simulink model "engine_test_bed"  (R2022b)
settings: Solver=FixedStepAuto  StartTime=0.0  StopTime=250  FixedStep=1e-3  RelTol=1e-3
InitFcn:
  | lqr_cont;
  | ref_calc;
values from neighbouring files (symbols this model uses):
  rpm = ones(1,3)    [ref_calc.m]
  torque = ones(1,3)    [ref_calc.m]
undefined symbols (not defined in the file or in its folder): K
settings Model: Creator=Cemil  LastModifiedBy=Cemil
settings SolverCC: AlgebraicLoopSolver=TrustRegion
settings DebuggingCC: UnconnectedInputMsg=warning  UnconnectedOutputMsg=warning  UnconnectedLineMsg=warning  SFMachineParentedDataDiag=warning
settings HardwareCC: ProdHWDeviceType=AMD->x86-64 (Windows64)
settings ModelReferenceCC: EnableRefExpFcnMdlSchedulingChecks=on
settings RTWCC: DLArmComputeVersion=19.05

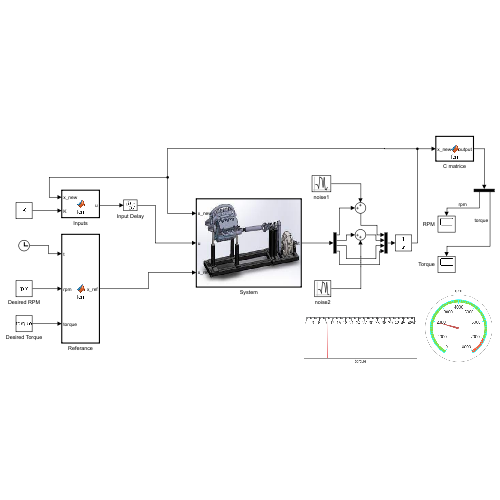
[thumbnail: Simulink's stored preview of the top-level diagram]
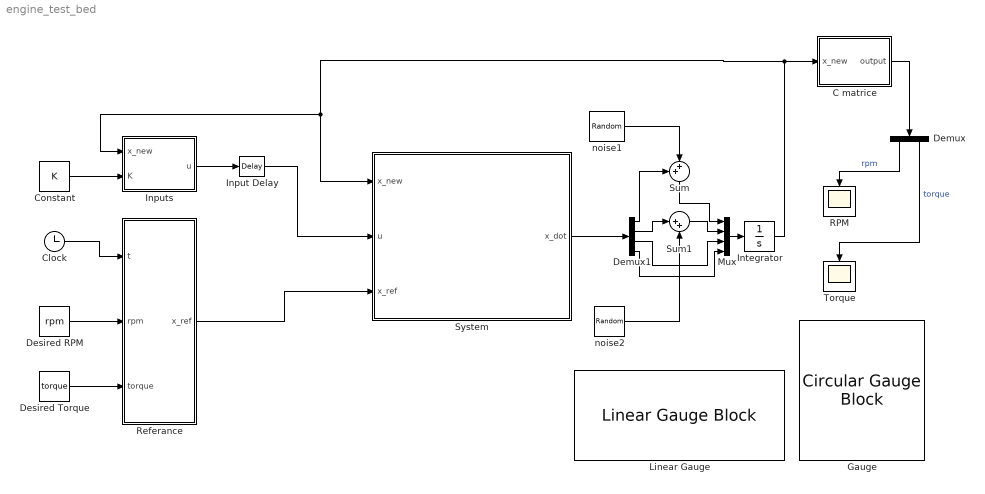
== system engine_test_bed ==
  C matrice : MATLAB Function  TreatAsAtomicUnit=on
  Clock : Clock
  Constant : Constant  Value=K  VectorParams1D=off
  Demux : Demux  Outputs=2
  Demux1 : Demux
  Desired RPM : Constant  Value=rpm  VectorParams1D=off
  Desired Torque : Constant  Value=torque  VectorParams1D=off
  Gauge : CircularGaugeBlock  ScaleMax=8000  TickInterval=1000
  Input Delay : TransportDelay  DelayTime=0.3
  Inputs : MATLAB Function  TreatAsAtomicUnit=on
  Integrator : Integrator  InitialCondition=[0;0;0;0]
  Linear Gauge : LinearGaugeBlock  LabelPosition=Bottom  ScaleMax=50
  Mux : Mux
  RPM : Scope
  Referance : MATLAB Function  TreatAsAtomicUnit=on
  Sum : Sum  Inputs=++|
  Sum1 : Sum  Inputs=|++
  System : MATLAB Function  TreatAsAtomicUnit=on
  Torque : Scope
  noise1 : RandomNumber  Mean=100  Variance=5  SampleTime=0.1  VectorParams1D=off
  noise2 : RandomNumber  Mean=1  SampleTime=0.1  VectorParams1D=off
  wires:
  Integrator/1 -> Inputs/1(x_new), System/1(x_new), C matrice/1(x_new)
  Inputs/1(u) -> Input Delay/1
  Constant/1 -> Inputs/2(K)
  Input Delay/1 -> System/2(u)
  Demux/2 -> Torque/1  "torque"
  Demux/1 -> RPM/1  "rpm"
  C matrice/1(output) -> Demux/1
  Clock/1 -> Referance/1(t)
  System/1(x_dot) -> Demux1/1
  Mux/1 -> Integrator/1
  Demux1/2 -> Sum1/1
  noise2/1 -> Sum1/2
  Sum1/1 -> Mux/2
  Demux1/3 -> Mux/3
  Demux1/4 -> Mux/4
  Demux1/1 -> Sum/1
  Sum/1 -> Mux/1
  noise1/1 -> Sum/2
  Desired RPM/1 -> Referance/2(rpm)
  Desired Torque/1 -> Referance/3(torque)
  Referance/1(x_ref) -> System/3(x_ref)

== matlab function engine_test_bed/Referance ==
  data: t input; x_ref output; rpm input; torque input
function x_ref = fcn(t,rpm,torque)



x_ref =[0; 0; rpm(1,1); torque(1,1)];


if t>25
    if t<65
        x_ref =[0; 0; rpm(1,2); torque(1,2)];       
    end
end

if t>90
    if t<125
        x_ref =[0; 0; rpm(1,3); torque(1,3)];       
    end
end

if t>150
    if t<190
        x_ref =[0; 0; rpm(1,2); torque(1,2)];       
    end
end

if t>220
    
        x_ref =[0; 0; rpm(1,2); torque(1,2)];       
    
end





    
    
    
    


end

== matlab function engine_test_bed/System ==
  data: x_new input; u input; x_dot output; x_ref input
function x_dot = fcn(x_new,u,x_ref)


A = [-1, 0;
     0, -1];
     

A_new = [A, zeros(2,1), zeros(2,1);
         1, 0, 0, 0;
         0, 1, 0, 0];

B_new = [1, 0;
         0, 1;
         0, 0;
         0, 0];

E_ref = [0, 0,0,0;
         0, 0,0,0;
         0, 0,-1,0;
         0,0,0, -1];

x_dot=A_new*x_new + B_new*u + E_ref*x_ref;
end

== matlab function engine_test_bed/Inputs ==
  data: x_new input; u output; K input
function u = fcn(x_new,K)


u= -K*x_new;
end

== matlab function engine_test_bed/C matrice ==
  data: x_new input; output output
function output = fcn(x_new)

output=zeros(2,1);
output(1,1) = 17.54*x_new(1)-3.18*x_new(2);
output(2,1) = 1.16*x_new(1)+2.32*x_new(2);


end
